simulink library "VISMODAL_MASTER"  (Simulink 8.6)
settings: Solver=VariableStepAuto  StartTime=0.0  StopTime=10.0  RelTol=1e-3
libraries: VIS_LIB x140, cdsFilt x34, cdsMuxMatrix x6, VISMODAL_MASTER x1
(part 4 of 5)

== system VISMODAL_MASTER/ITMY/SUM_GAS ==
  note: #DAQ Channels
      |
      | M1_OUT 256
      | M2_OUT 256
      | M3_OUT 256
      | M4_OUT 256
      | M5_OUT 256
  M1_IN : Inport
  M2_IN : Inport  Port=2
  M3_IN : Inport  Port=3
  M4_IN : Inport  Port=4
  M5_IN : Inport  Port=5
  M1 : cdsFilt/Subsystem  Tag=cdsFilt  Description=|
      | Purpose:                                                                                                                                                                                                                                  
      | Standard CDS IIR filter module.                                                                                                                                                                                                           
      |                                                                                                                                                                                                                                           
      | Operation:                                                                                                                                                                                                                                
      | Consists of 10 second order section IIR filters, plus a ramped gain stage. In FE code, also provides pre-defined test points and excitation channel inputs. The filter coefficients are defined in the LIGO system using the 'foton' tool.
      |                                                                                                                                                                                                                                           
      | Usage:                                                                                                                                                                                                                                    
      | Name the part with the desired filter module name.
      settings: AttributesFormatString=%<Tag>
  M2 : cdsFilt/Subsystem  Tag=cdsFilt  Description=|
      | Purpose:                                                                                                                                                                                                                                  
      | Standard CDS IIR filter module.                                                                                                                                                                                                           
      |                                                                                                                                                                                                                                           
      | Operation:                                                                                                                                                                                                                                
      | Consists of 10 second order section IIR filters, plus a ramped gain stage. In FE code, also provides pre-defined test points and excitation channel inputs. The filter coefficients are defined in the LIGO system using the 'foton' tool.
      |                                                                                                                                                                                                                                           
      | Usage:                                                                                                                                                                                                                                    
      | Name the part with the desired filter module name.
      settings: AttributesFormatString=%<Tag>
  M3 : cdsFilt/Subsystem  Tag=cdsFilt  Description=|
      | Purpose:                                                                                                                                                                                                                                  
      | Standard CDS IIR filter module.                                                                                                                                                                                                           
      |                                                                                                                                                                                                                                           
      | Operation:                                                                                                                                                                                                                                
      | Consists of 10 second order section IIR filters, plus a ramped gain stage. In FE code, also provides pre-defined test points and excitation channel inputs. The filter coefficients are defined in the LIGO system using the 'foton' tool.
      |                                                                                                                                                                                                                                           
      | Usage:                                                                                                                                                                                                                                    
      | Name the part with the desired filter module name.
      settings: AttributesFormatString=%<Tag>
  M4 : cdsFilt/Subsystem  Tag=cdsFilt  Description=|
      | Purpose:                                                                                                                                                                                                                                  
      | Standard CDS IIR filter module.                                                                                                                                                                                                           
      |                                                                                                                                                                                                                                           
      | Operation:                                                                                                                                                                                                                                
      | Consists of 10 second order section IIR filters, plus a ramped gain stage. In FE code, also provides pre-defined test points and excitation channel inputs. The filter coefficients are defined in the LIGO system using the 'foton' tool.
      |                                                                                                                                                                                                                                           
      | Usage:                                                                                                                                                                                                                                    
      | Name the part with the desired filter module name.
      settings: AttributesFormatString=%<Tag>
  M5 : cdsFilt/Subsystem  Tag=cdsFilt  Description=|
      | Purpose:                                                                                                                                                                                                                                  
      | Standard CDS IIR filter module.                                                                                                                                                                                                           
      |                                                                                                                                                                                                                                           
      | Operation:                                                                                                                                                                                                                                
      | Consists of 10 second order section IIR filters, plus a ramped gain stage. In FE code, also provides pre-defined test points and excitation channel inputs. The filter coefficients are defined in the LIGO system using the 'foton' tool.
      |                                                                                                                                                                                                                                           
      | Usage:                                                                                                                                                                                                                                    
      | Name the part with the desired filter module name.
      settings: AttributesFormatString=%<Tag>
  M1_OUT : Outport
  M2_OUT : Outport  Port=2
  M3_OUT : Outport  Port=3
  M4_OUT : Outport  Port=4
  M5_OUT : Outport  Port=5
  wires:
  M3/1 -> M3_OUT/1
  M2/1 -> M2_OUT/1
  M4/1 -> M4_OUT/1
  M5/1 -> M5_OUT/1
  M1/1 -> M1_OUT/1
  M1_IN/1 -> M1/1
  M2_IN/1 -> M2/1
  M3_IN/1 -> M3/1
  M4_IN/1 -> M4/1
  M5_IN/1 -> M5/1

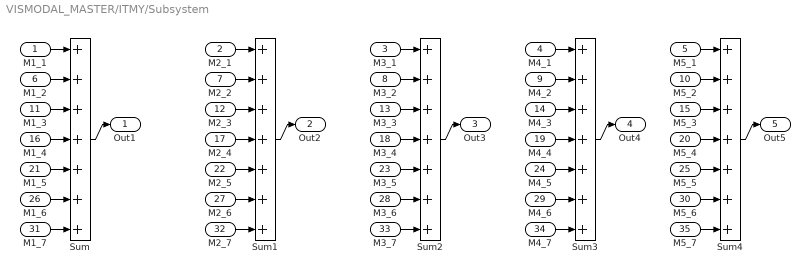
== system VISMODAL_MASTER/ITMY/Subsystem ==
  M1_1 : Inport
  M2_1 : Inport  Port=2
  M3_1 : Inport  Port=3
  M4_1 : Inport  Port=4
  M5_1 : Inport  Port=5
  M1_2 : Inport  Port=6
  M2_2 : Inport  Port=7
  M3_2 : Inport  Port=8
  M4_2 : Inport  Port=9
  M5_2 : Inport  Port=10
  M1_3 : Inport  Port=11
  M2_3 : Inport  Port=12
  M3_3 : Inport  Port=13
  M4_3 : Inport  Port=14
  M5_3 : Inport  Port=15
  M1_4 : Inport  Port=16
  M2_4 : Inport  Port=17
  M3_4 : Inport  Port=18
  M4_4 : Inport  Port=19
  M5_4 : Inport  Port=20
  M1_5 : Inport  Port=21
  M2_5 : Inport  Port=22
  M3_5 : Inport  Port=23
  M4_5 : Inport  Port=24
  M5_5 : Inport  Port=25
  M1_6 : Inport  Port=26
  M2_6 : Inport  Port=27
  M3_6 : Inport  Port=28
  M4_6 : Inport  Port=29
  M5_6 : Inport  Port=30
  M1_7 : Inport  Port=31
  M2_7 : Inport  Port=32
  M3_7 : Inport  Port=33
  M4_7 : Inport  Port=34
  M5_7 : Inport  Port=35
  Sum{,1..4} (5 alike) : Sum  Inputs=+++++++
  Out1 : Outport
  Out2 : Outport  Port=2
  Out3 : Outport  Port=3
  Out4 : Outport  Port=4
  Out5 : Outport  Port=5
  wires:
  M1_1/1 -> Sum/1
  Sum/1 -> Out1/1
  M2_1/1 -> Sum1/1
  Sum1/1 -> Out2/1
  M3_1/1 -> Sum2/1
  Sum2/1 -> Out3/1
  M4_1/1 -> Sum3/1
  Sum3/1 -> Out4/1
  M5_1/1 -> Sum4/1
  Sum4/1 -> Out5/1
  M1_2/1 -> Sum/2
  M2_2/1 -> Sum1/2
  M3_2/1 -> Sum2/2
  M4_2/1 -> Sum3/2
  M5_2/1 -> Sum4/2
  M1_3/1 -> Sum/3
  M2_3/1 -> Sum1/3
  M3_3/1 -> Sum2/3
  M4_3/1 -> Sum3/3
  M5_3/1 -> Sum4/3
  M1_4/1 -> Sum/4
  M2_4/1 -> Sum1/4
  M3_4/1 -> Sum2/4
  M4_4/1 -> Sum3/4
  M5_4/1 -> Sum4/4
  M1_5/1 -> Sum/5
  M2_5/1 -> Sum1/5
  M3_5/1 -> Sum2/5
  M4_5/1 -> Sum3/5
  M5_5/1 -> Sum4/5
  M1_6/1 -> Sum/6
  M2_6/1 -> Sum1/6
  M3_6/1 -> Sum2/6
  M4_6/1 -> Sum3/6
  M5_6/1 -> Sum4/6
  M5_7/1 -> Sum4/7
  M4_7/1 -> Sum3/7
  M3_7/1 -> Sum2/7
  M2_7/1 -> Sum1/7
  M1_7/1 -> Sum/7

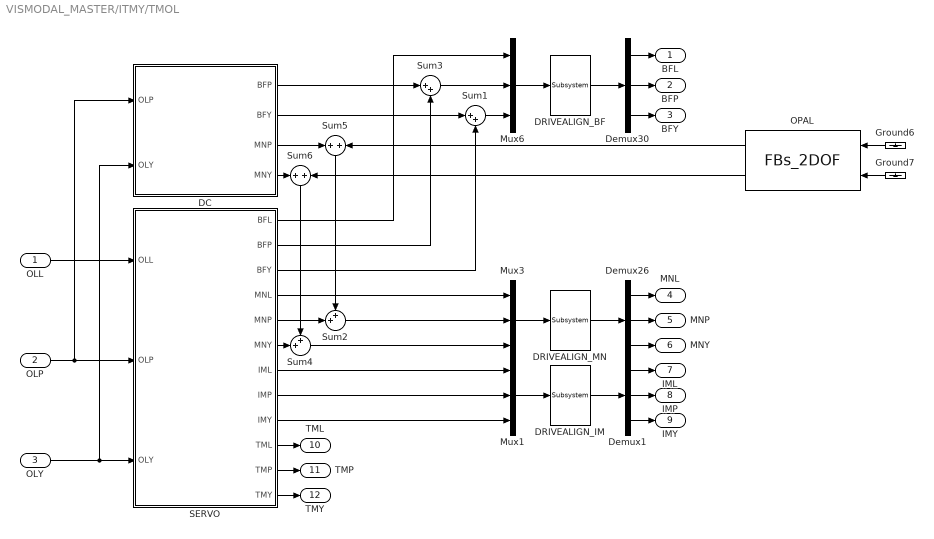
== system VISMODAL_MASTER/ITMY/TMOL ==
  OLL : Inport
  OLP : Inport  Port=2
  OLY : Inport  Port=3
  DC : Subsystem
  DRIVEALIGN_BF : cdsMuxMatrix/Subsystem  Tag=cdsMuxMatrix  Description=Any size matrix. Inputs and outputs must be connected using Mux and Demux parts.
      settings: AttributesFormatString=%<Tag>
  DRIVEALIGN_IM : cdsMuxMatrix/Subsystem  Tag=cdsMuxMatrix  Description=Any size matrix. Inputs and outputs must be connected using Mux and Demux parts.
      settings: AttributesFormatString=%<Tag>
  DRIVEALIGN_MN : cdsMuxMatrix/Subsystem  Tag=cdsMuxMatrix  Description=Any size matrix. Inputs and outputs must be connected using Mux and Demux parts.
      settings: AttributesFormatString=%<Tag>
  Demux1 : Demux  Outputs=3
  Demux26 : Demux  Outputs=3
  Demux30 : Demux  Outputs=3
  Ground6 : Ground
  Ground7 : Ground
  Mux1 : Mux  Inputs=3
  Mux3 : Mux  Inputs=3
  Mux6 : Mux  Inputs=3
  OPAL : VIS_LIB/UTILs/FBs_2DOF
  SERVO : Subsystem
  Sum1 : Sum  Inputs=|++
  Sum2 : Sum  Inputs=++|
  Sum3 : Sum  Inputs=|++
  Sum4 : Sum  Inputs=++|
  Sum5 : Sum
  Sum6 : Sum
  BFL : Outport
  BFP : Outport  Port=2
  BFY : Outport  Port=3
  MNL : Outport  Port=4
  MNP : Outport  Port=5
  MNY : Outport  Port=6
  IML : Outport  Port=7
  IMP : Outport  Port=8
  IMY : Outport  Port=9
  TML : Outport  Port=10
  TMP : Outport  Port=11
  TMY : Outport  Port=12
  wires:
  Mux3/1 -> DRIVEALIGN_MN/1
  DRIVEALIGN_MN/1 -> Demux26/1
  Mux6/1 -> DRIVEALIGN_BF/1
  DRIVEALIGN_BF/1 -> Demux30/1
  Demux30/1 -> BFL/1
  Demux30/2 -> BFP/1
  Demux26/1 -> MNL/1
  Demux26/2 -> MNP/1
  SERVO/1(BFL) -> Mux6/1
  Sum3/1 -> Mux6/2
  SERVO/2(BFP) -> Sum3/2
  DC/1(BFP) -> Sum3/1
  Sum1/1 -> Mux6/3
  DC/2(BFY) -> Sum1/1
  SERVO/3(BFY) -> Sum1/2
  SERVO/4(MNL) -> Mux3/1
  Sum2/1 -> Mux3/2
  SERVO/5(MNP) -> Sum2/2
  SERVO/6(MNY) -> Sum4/2
  Sum4/1 -> Mux3/3
  Demux30/3 -> BFY/1
  Demux26/3 -> MNY/1
  Mux1/1 -> DRIVEALIGN_IM/1
  DRIVEALIGN_IM/1 -> Demux1/1
  Demux1/1 -> IML/1
  Demux1/2 -> IMP/1
  SERVO/7(IML) -> Mux1/1
  SERVO/8(IMP) -> Mux1/2
  SERVO/9(IMY) -> Mux1/3
  Demux1/3 -> IMY/1
  SERVO/10(TML) -> TML/1
  SERVO/11(TMP) -> TMP/1
  SERVO/12(TMY) -> TMY/1
  DC/3(MNP) -> Sum5/1
  Sum5/1 -> Sum2/1
  DC/4(MNY) -> Sum6/1
  Sum6/1 -> Sum4/1
  OLL/1 -> SERVO/1(OLL)
  OLP/1 -> DC/1(OLP), SERVO/2(OLP)
  OLY/1 -> DC/2(OLY), SERVO/3(OLY)
  Ground6/1 -> OPAL/1
  Ground7/1 -> OPAL/2
  OPAL/2 -> Sum6/2
  OPAL/1 -> Sum5/2

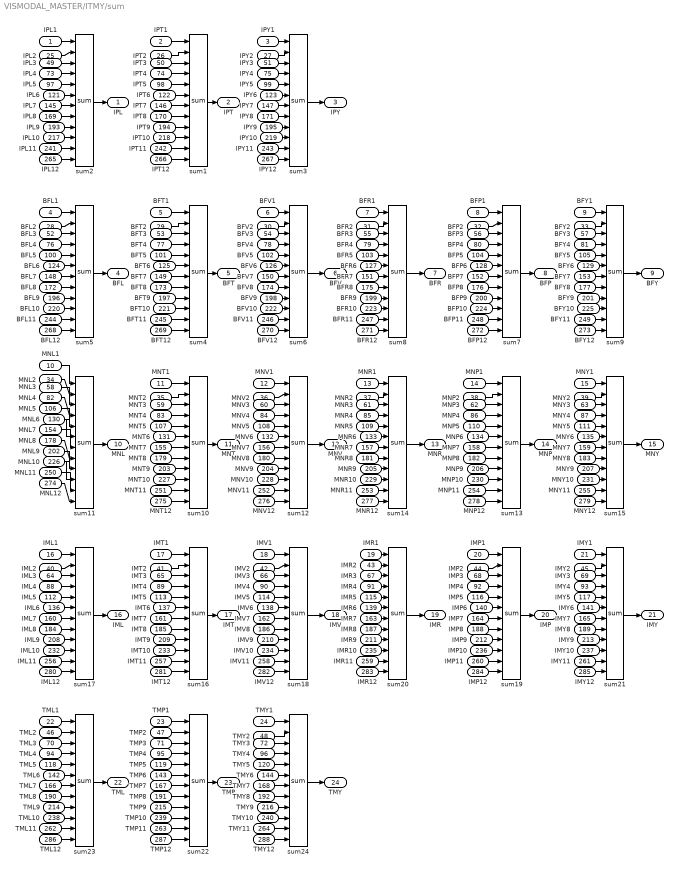
== system VISMODAL_MASTER/ITMY/sum ==
  IPL1 : Inport
  IPT1 : Inport  Port=2
  IPY1 : Inport  Port=3
  BFL1 : Inport  Port=4
  BFT1 : Inport  Port=5
  BFV1 : Inport  Port=6
  BFR1 : Inport  Port=7
  BFP1 : Inport  Port=8
  BFY1 : Inport  Port=9
  MNL1 : Inport  Port=10
  MNT1 : Inport  Port=11
  MNV1 : Inport  Port=12
  MNR1 : Inport  Port=13
  MNP1 : Inport  Port=14
  MNY1 : Inport  Port=15
  IML1 : Inport  Port=16
  IMT1 : Inport  Port=17
  IMV1 : Inport  Port=18
  IMR1 : Inport  Port=19
  IMP1 : Inport  Port=20
  IMY1 : Inport  Port=21
  TML1 : Inport  Port=22
  TMP1 : Inport  Port=23
  TMY1 : Inport  Port=24
  IPL2 : Inport  Port=25
  IPT2 : Inport  Port=26
  IPY2 : Inport  Port=27
  BFL2 : Inport  Port=28
  BFT2 : Inport  Port=29
  BFV2 : Inport  Port=30
  BFR2 : Inport  Port=31
  BFP2 : Inport  Port=32
  BFY2 : Inport  Port=33
  MNL2 : Inport  Port=34
  MNT2 : Inport  Port=35
  MNV2 : Inport  Port=36
  MNR2 : Inport  Port=37
  MNP2 : Inport  Port=38
  MNY2 : Inport  Port=39
  IML2 : Inport  Port=40
  IMT2 : Inport  Port=41
  IMV2 : Inport  Port=42
  IMR2 : Inport  Port=43
  IMP2 : Inport  Port=44
  IMY2 : Inport  Port=45
  TML2 : Inport  Port=46
  TMP2 : Inport  Port=47
  TMY2 : Inport  Port=48
  IPL3 : Inport  Port=49
  IPT3 : Inport  Port=50
  IPY3 : Inport  Port=51
  BFL3 : Inport  Port=52
  BFT3 : Inport  Port=53
  BFV3 : Inport  Port=54
  BFR3 : Inport  Port=55
  BFP3 : Inport  Port=56
  BFY3 : Inport  Port=57
  MNL3 : Inport  Port=58
  MNT3 : Inport  Port=59
  MNV3 : Inport  Port=60
  MNR3 : Inport  Port=61
  MNP3 : Inport  Port=62
  MNY3 : Inport  Port=63
  IML3 : Inport  Port=64
  IMT3 : Inport  Port=65
  IMV3 : Inport  Port=66
  IMR3 : Inport  Port=67
  IMP3 : Inport  Port=68
  IMY3 : Inport  Port=69
  TML3 : Inport  Port=70
  TMP3 : Inport  Port=71
  TMY3 : Inport  Port=72
  IPL4 : Inport  Port=73
  IPT4 : Inport  Port=74
  IPY4 : Inport  Port=75
  BFL4 : Inport  Port=76
  BFT4 : Inport  Port=77
  BFV4 : Inport  Port=78
  BFR4 : Inport  Port=79
  BFP4 : Inport  Port=80
  BFY4 : Inport  Port=81
  MNL4 : Inport  Port=82
  MNT4 : Inport  Port=83
  MNV4 : Inport  Port=84
  MNR4 : Inport  Port=85
  MNP4 : Inport  Port=86
  MNY4 : Inport  Port=87
  IML4 : Inport  Port=88
  IMT4 : Inport  Port=89
  IMV4 : Inport  Port=90
  IMR4 : Inport  Port=91
  IMP4 : Inport  Port=92
  IMY4 : Inport  Port=93
  TML4 : Inport  Port=94
  TMP4 : Inport  Port=95
  TMY4 : Inport  Port=96
  IPL5 : Inport  Port=97
  IPT5 : Inport  Port=98
  IPY5 : Inport  Port=99
  BFL5 : Inport  Port=100
  BFT5 : Inport  Port=101
  BFV5 : Inport  Port=102
  BFR5 : Inport  Port=103
  BFP5 : Inport  Port=104
  BFY5 : Inport  Port=105
  MNL5 : Inport  Port=106
  MNT5 : Inport  Port=107
  MNV5 : Inport  Port=108
  MNR5 : Inport  Port=109
  MNP5 : Inport  Port=110
  MNY5 : Inport  Port=111
  IML5 : Inport  Port=112
  IMT5 : Inport  Port=113
  IMV5 : Inport  Port=114
  IMR5 : Inport  Port=115
  IMP5 : Inport  Port=116
  IMY5 : Inport  Port=117
  TML5 : Inport  Port=118
  TMP5 : Inport  Port=119
  TMY5 : Inport  Port=120
  IPL6 : Inport  Port=121
  IPT6 : Inport  Port=122
  IPY6 : Inport  Port=123
  BFL6 : Inport  Port=124
  BFT6 : Inport  Port=125
  BFV6 : Inport  Port=126
  BFR6 : Inport  Port=127
  BFP6 : Inport  Port=128
  BFY6 : Inport  Port=129
  MNL6 : Inport  Port=130
  MNT6 : Inport  Port=131
  MNV6 : Inport  Port=132
  MNR6 : Inport  Port=133
  MNP6 : Inport  Port=134
  MNY6 : Inport  Port=135
  IML6 : Inport  Port=136
  IMT6 : Inport  Port=137
  IMV6 : Inport  Port=138
  IMR6 : Inport  Port=139
  IMP6 : Inport  Port=140
  IMY6 : Inport  Port=141
  TML6 : Inport  Port=142
  TMP6 : Inport  Port=143
  TMY6 : Inport  Port=144
  IPL7 : Inport  Port=145
  IPT7 : Inport  Port=146
  IPY7 : Inport  Port=147
  BFL7 : Inport  Port=148
  BFT7 : Inport  Port=149
  BFV7 : Inport  Port=150
  BFR7 : Inport  Port=151
  BFP7 : Inport  Port=152
  BFY7 : Inport  Port=153
  MNL7 : Inport  Port=154
  MNT7 : Inport  Port=155
  MNV7 : Inport  Port=156
  MNR7 : Inport  Port=157
  MNP7 : Inport  Port=158
  MNY7 : Inport  Port=159
  IML7 : Inport  Port=160
  IMT7 : Inport  Port=161
  IMV7 : Inport  Port=162
  IMR7 : Inport  Port=163
  IMP7 : Inport  Port=164
  IMY7 : Inport  Port=165
  TML7 : Inport  Port=166
  TMP7 : Inport  Port=167
  TMY7 : Inport  Port=168
  IPL8 : Inport  Port=169
  IPT8 : Inport  Port=170
  IPY8 : Inport  Port=171
  BFL8 : Inport  Port=172
  BFT8 : Inport  Port=173
  BFV8 : Inport  Port=174
  BFR8 : Inport  Port=175
  BFP8 : Inport  Port=176
  BFY8 : Inport  Port=177
  MNL8 : Inport  Port=178
  MNT8 : Inport  Port=179
  MNV8 : Inport  Port=180
  MNR8 : Inport  Port=181
  MNP8 : Inport  Port=182
  MNY8 : Inport  Port=183
  IML8 : Inport  Port=184
  IMT8 : Inport  Port=185
  IMV8 : Inport  Port=186
  IMR8 : Inport  Port=187
  IMP8 : Inport  Port=188
  IMY8 : Inport  Port=189
  TML8 : Inport  Port=190
  TMP8 : Inport  Port=191
  TMY8 : Inport  Port=192
  IPL9 : Inport  Port=193
  IPT9 : Inport  Port=194
  IPY9 : Inport  Port=195
  BFL9 : Inport  Port=196
  BFT9 : Inport  Port=197
  BFV9 : Inport  Port=198
  BFR9 : Inport  Port=199
  BFP9 : Inport  Port=200
  BFY9 : Inport  Port=201
  MNL9 : Inport  Port=202
  MNT9 : Inport  Port=203
  MNV9 : Inport  Port=204
  MNR9 : Inport  Port=205
  MNP9 : Inport  Port=206
  MNY9 : Inport  Port=207
  IML9 : Inport  Port=208
  IMT9 : Inport  Port=209
  IMV9 : Inport  Port=210
  IMR9 : Inport  Port=211
  IMP9 : Inport  Port=212
  IMY9 : Inport  Port=213
  TML9 : Inport  Port=214
  TMP9 : Inport  Port=215
  TMY9 : Inport  Port=216
  IPL10 : Inport  Port=217
  IPT10 : Inport  Port=218
  IPY10 : Inport  Port=219
  BFL10 : Inport  Port=220
  BFT10 : Inport  Port=221
  BFV10 : Inport  Port=222
  BFR10 : Inport  Port=223
  BFP10 : Inport  Port=224
  BFY10 : Inport  Port=225
  MNL10 : Inport  Port=226
  MNT10 : Inport  Port=227
  MNV10 : Inport  Port=228
  MNR10 : Inport  Port=229
  MNP10 : Inport  Port=230
  MNY10 : Inport  Port=231
  IML10 : Inport  Port=232
  IMT10 : Inport  Port=233
  IMV10 : Inport  Port=234
  IMR10 : Inport  Port=235
  IMP10 : Inport  Port=236
  IMY10 : Inport  Port=237
  TML10 : Inport  Port=238
  TMP10 : Inport  Port=239
  TMY10 : Inport  Port=240
  IPL11 : Inport  Port=241
  IPT11 : Inport  Port=242
  IPY11 : Inport  Port=243
  BFL11 : Inport  Port=244
  BFT11 : Inport  Port=245
  BFV11 : Inport  Port=246
  BFR11 : Inport  Port=247
  BFP11 : Inport  Port=248
  BFY11 : Inport  Port=249
  MNL11 : Inport  Port=250
  MNT11 : Inport  Port=251
  MNV11 : Inport  Port=252
  MNR11 : Inport  Port=253
  MNP11 : Inport  Port=254
  MNY11 : Inport  Port=255
  IML11 : Inport  Port=256
  IMT11 : Inport  Port=257
  IMV11 : Inport  Port=258
  IMR11 : Inport  Port=259
  IMP11 : Inport  Port=260
  IMY11 : Inport  Port=261
  TML11 : Inport  Port=262
  TMP11 : Inport  Port=263
  TMY11 : Inport  Port=264
  IPL12 : Inport  Port=265
  IPT12 : Inport  Port=266
  IPY12 : Inport  Port=267
  BFL12 : Inport  Port=268
  BFT12 : Inport  Port=269
  BFV12 : Inport  Port=270
  BFR12 : Inport  Port=271
  BFP12 : Inport  Port=272
  BFY12 : Inport  Port=273
  MNL12 : Inport  Port=274
  MNT12 : Inport  Port=275
  MNV12 : Inport  Port=276
  MNR12 : Inport  Port=277
  MNP12 : Inport  Port=278
  MNY12 : Inport  Port=279
  IML12 : Inport  Port=280
  IMT12 : Inport  Port=281
  IMV12 : Inport  Port=282
  IMR12 : Inport  Port=283
  IMP12 : Inport  Port=284
  IMY12 : Inport  Port=285
  TML12 : Inport  Port=286
  TMP12 : Inport  Port=287
  TMY12 : Inport  Port=288
  sum{1..24} (24 alike) : VIS_LIB/MODAL/sum
  IPL : Outport
  IPT : Outport  Port=2
  IPY : Outport  Port=3
  BFL : Outport  Port=4
  BFT : Outport  Port=5
  BFV : Outport  Port=6
  BFR : Outport  Port=7
  BFP : Outport  Port=8
  BFY : Outport  Port=9
  MNL : Outport  Port=10
  MNT : Outport  Port=11
  MNV : Outport  Port=12
  MNR : Outport  Port=13
  MNP : Outport  Port=14
  MNY : Outport  Port=15
  IML : Outport  Port=16
  IMT : Outport  Port=17
  IMV : Outport  Port=18
  IMR : Outport  Port=19
  IMP : Outport  Port=20
  IMY : Outport  Port=21
  TML : Outport  Port=22
  TMP : Outport  Port=23
  TMY : Outport  Port=24
  wires:
  IPT2/1 -> sum1/2
  IPT1/1 -> sum1/1
  IPL1/1 -> sum2/1
  IPL2/1 -> sum2/2
  IPY1/1 -> sum3/1
  IPY2/1 -> sum3/2
  BFT1/1 -> sum4/1
  BFT2/1 -> sum4/2
  BFL1/1 -> sum5/1
  BFL2/1 -> sum5/2
  BFV1/1 -> sum6/1
  BFV2/1 -> sum6/2
  BFR1/1 -> sum8/1
  BFR2/1 -> sum8/2
  BFP1/1 -> sum7/1
  BFP2/1 -> sum7/2
  BFY1/1 -> sum9/1
  BFY2/1 -> sum9/2
  MNT1/1 -> sum10/1
  MNT2/1 -> sum10/2
  MNL1/1 -> sum11/1
  MNL2/1 -> sum11/2
  MNV1/1 -> sum12/1
  MNV2/1 -> sum12/2
  MNR1/1 -> sum14/1
  MNR2/1 -> sum14/2
  MNP1/1 -> sum13/1
  MNP2/1 -> sum13/2
  MNY1/1 -> sum15/1
  MNY2/1 -> sum15/2
  IMT1/1 -> sum16/1
  IMT2/1 -> sum16/2
  IML1/1 -> sum17/1
  IML2/1 -> sum17/2
  IMV1/1 -> sum18/1
  IMV2/1 -> sum18/2
  IMP1/1 -> sum19/1
  IMP2/1 -> sum19/2
  IMY1/1 -> sum21/1
  IMY2/1 -> sum21/2
  TML2/1 -> sum23/2
  TML1/1 -> sum23/1
  TMP1/1 -> sum22/1
  TMP2/1 -> sum22/2
  TMY1/1 -> sum24/1
  TMY2/1 -> sum24/2
  sum24/1 -> TMY/1
  sum22/1 -> TMP/1
  sum23/1 -> TML/1
  sum17/1 -> IML/1
  sum16/1 -> IMT/1
  sum18/1 -> IMV/1
  sum20/1 -> IMR/1
  sum19/1 -> IMP/1
  sum21/1 -> IMY/1
  sum3/1 -> IPY/1
  sum1/1 -> IPT/1
  sum4/1 -> BFT/1
  sum6/1 -> BFV/1
  sum12/1 -> MNV/1
  sum14/1 -> MNR/1
  sum8/1 -> BFR/1
  sum7/1 -> BFP/1
  sum9/1 -> BFY/1
  sum15/1 -> MNY/1
  sum13/1 -> MNP/1
  sum10/1 -> MNT/1
  sum11/1 -> MNL/1
  sum5/1 -> BFL/1
  sum2/1 -> IPL/1
  IPT3/1 -> sum1/3
  IPL3/1 -> sum2/3
  IPY3/1 -> sum3/3
  BFT3/1 -> sum4/3
  BFL3/1 -> sum5/3
  BFV3/1 -> sum6/3
  BFR3/1 -> sum8/3
  BFP3/1 -> sum7/3
  BFY3/1 -> sum9/3
  MNT3/1 -> sum10/3
  MNL3/1 -> sum11/3
  MNV3/1 -> sum12/3
  MNR3/1 -> sum14/3
  MNP3/1 -> sum13/3
  MNY3/1 -> sum15/3
  IMT3/1 -> sum16/3
  IML3/1 -> sum17/3
  IMV3/1 -> sum18/3
  IMP3/1 -> sum19/3
  IMY3/1 -> sum21/3
  TML3/1 -> sum23/3
  TMP3/1 -> sum22/3
  TMY3/1 -> sum24/3
  IPT4/1 -> sum1/4
  IPL4/1 -> sum2/4
  IPY4/1 -> sum3/4
  BFT4/1 -> sum4/4
  BFL4/1 -> sum5/4
  BFV4/1 -> sum6/4
  BFR4/1 -> sum8/4
  BFP4/1 -> sum7/4
  BFY4/1 -> sum9/4
  MNT4/1 -> sum10/4
  MNL4/1 -> sum11/4
  MNV4/1 -> sum12/4
  MNR4/1 -> sum14/4
  MNP4/1 -> sum13/4
  MNY4/1 -> sum15/4
  IMT4/1 -> sum16/4
  IML4/1 -> sum17/4
  IMV4/1 -> sum18/4
  IMP4/1 -> sum19/4
  IMY4/1 -> sum21/4
  TML4/1 -> sum23/4
  TMP4/1 -> sum22/4
  TMY4/1 -> sum24/4
  IPT5/1 -> sum1/5
  IPL5/1 -> sum2/5
  IPY5/1 -> sum3/5
  BFT5/1 -> sum4/5
  BFL5/1 -> sum5/5
  BFV5/1 -> sum6/5
  BFR5/1 -> sum8/5
  BFP5/1 -> sum7/5
  BFY5/1 -> sum9/5
  MNT5/1 -> sum10/5
  MNL5/1 -> sum11/5
  MNV5/1 -> sum12/5
  MNR5/1 -> sum14/5
  MNP5/1 -> sum13/5
  MNY5/1 -> sum15/5
  IMT5/1 -> sum16/5
  IML5/1 -> sum17/5
  IMV5/1 -> sum18/5
  IMP5/1 -> sum19/5
  IMY5/1 -> sum21/5
  TML5/1 -> sum23/5
  TMP5/1 -> sum22/5
  TMY5/1 -> sum24/5
  IPT6/1 -> sum1/6
  IPL6/1 -> sum2/6
  IPY6/1 -> sum3/6
  BFT6/1 -> sum4/6
  BFL6/1 -> sum5/6
  BFV6/1 -> sum6/6
  BFR6/1 -> sum8/6
  BFP6/1 -> sum7/6
  BFY6/1 -> sum9/6
  MNT6/1 -> sum10/6
  MNL6/1 -> sum11/6
  MNV6/1 -> sum12/6
  MNR6/1 -> sum14/6
  MNP6/1 -> sum13/6
  MNY6/1 -> sum15/6
  IMT6/1 -> sum16/6
  IML6/1 -> sum17/6
  IMV6/1 -> sum18/6
  IMP6/1 -> sum19/6
  IMY6/1 -> sum21/6
  TML6/1 -> sum23/6
  TMP6/1 -> sum22/6
  TMY6/1 -> sum24/6
  IPT7/1 -> sum1/7
  IPL7/1 -> sum2/7
  IPY7/1 -> sum3/7
  BFT7/1 -> sum4/7
  BFL7/1 -> sum5/7
  BFV7/1 -> sum6/7
  BFR7/1 -> sum8/7
  BFP7/1 -> sum7/7
  BFY7/1 -> sum9/7
  MNT7/1 -> sum10/7
  MNL7/1 -> sum11/7
  MNV7/1 -> sum12/7
  MNR7/1 -> sum14/7
  MNP7/1 -> sum13/7
  MNY7/1 -> sum15/7
  IMT7/1 -> sum16/7
  IML7/1 -> sum17/7
  IMV7/1 -> sum18/7
  IMP7/1 -> sum19/7
  IMY7/1 -> sum21/7
  TML7/1 -> sum23/7
  TMP7/1 -> sum22/7
  TMY7/1 -> sum24/7
  IPT8/1 -> sum1/8
  IPL8/1 -> sum2/8
  IPY8/1 -> sum3/8
  BFT8/1 -> sum4/8
  BFL8/1 -> sum5/8
  BFV8/1 -> sum6/8
  BFR8/1 -> sum8/8
  BFP8/1 -> sum7/8
  BFY8/1 -> sum9/8
  MNT8/1 -> sum10/8
  MNL8/1 -> sum11/8
  MNV8/1 -> sum12/8
  MNR8/1 -> sum14/8
  MNP8/1 -> sum13/8
  MNY8/1 -> sum15/8
  IMT8/1 -> sum16/8
  IML8/1 -> sum17/8
  IMV8/1 -> sum18/8
  IMP8/1 -> sum19/8
  IMY8/1 -> sum21/8
  TML8/1 -> sum23/8
  TMP8/1 -> sum22/8
  TMY8/1 -> sum24/8
  IPT9/1 -> sum1/9
  IPL9/1 -> sum2/9
  IPY9/1 -> sum3/9
  BFT9/1 -> sum4/9
  BFL9/1 -> sum5/9
  BFV9/1 -> sum6/9
  BFR9/1 -> sum8/9
  BFP9/1 -> sum7/9
  BFY9/1 -> sum9/9
  MNT9/1 -> sum10/9
  MNL9/1 -> sum11/9
  MNV9/1 -> sum12/9
  MNR9/1 -> sum14/9
  MNP9/1 -> sum13/9
  MNY9/1 -> sum15/9
  IMT9/1 -> sum16/9
  IML9/1 -> sum17/9
  IMV9/1 -> sum18/9
  IMP9/1 -> sum19/9
  IMY9/1 -> sum21/9
  TML9/1 -> sum23/9
  TMP9/1 -> sum22/9
  TMY9/1 -> sum24/9
  IPT10/1 -> sum1/10
  IPL10/1 -> sum2/10
  IPY10/1 -> sum3/10
  BFT10/1 -> sum4/10
  BFL10/1 -> sum5/10
  BFV10/1 -> sum6/10
  BFR10/1 -> sum8/10
  BFP10/1 -> sum7/10
  BFY10/1 -> sum9/10
  MNT10/1 -> sum10/10
  MNL10/1 -> sum11/10
  MNV10/1 -> sum12/10
  MNR10/1 -> sum14/10
  MNP10/1 -> sum13/10
  MNY10/1 -> sum15/10
  IMT10/1 -> sum16/10
  IML10/1 -> sum17/10
  IMV10/1 -> sum18/10
  IMP10/1 -> sum19/10
  IMY10/1 -> sum21/10
  TML10/1 -> sum23/10
  TMP10/1 -> sum22/10
  TMY10/1 -> sum24/10
  IPT11/1 -> sum1/11
  IPL11/1 -> sum2/11
  IPY11/1 -> sum3/11
  BFT11/1 -> sum4/11
  BFL11/1 -> sum5/11
  BFV11/1 -> sum6/11
  BFR11/1 -> sum8/11
  BFP11/1 -> sum7/11
  BFY11/1 -> sum9/11
  MNT11/1 -> sum10/11
  MNL11/1 -> sum11/11
  MNV11/1 -> sum12/11
  MNR11/1 -> sum14/11
  MNP11/1 -> sum13/11
  MNY11/1 -> sum15/11
  IMT11/1 -> sum16/11
  IML11/1 -> sum17/11
  IMV11/1 -> sum18/11
  IMP11/1 -> sum19/11
  IMY11/1 -> sum21/11
  TML11/1 -> sum23/11
  TMP11/1 -> sum22/11
  TMY11/1 -> sum24/11
  IPT12/1 -> sum1/12
  IPL12/1 -> sum2/12
  IPY12/1 -> sum3/12
  BFT12/1 -> sum4/12
  BFL12/1 -> sum5/12
  BFV12/1 -> sum6/12
  BFR12/1 -> sum8/12
  BFP12/1 -> sum7/12
  BFY12/1 -> sum9/12
  MNT12/1 -> sum10/12
  MNL12/1 -> sum11/12
  MNV12/1 -> sum12/12
  MNR12/1 -> sum14/12
  MNP12/1 -> sum13/12
  MNY12/1 -> sum15/12
  IMT12/1 -> sum16/12
  IML12/1 -> sum17/12
  IMV12/1 -> sum18/12
  IMP12/1 -> sum19/12
  IMY12/1 -> sum21/12
  TML12/1 -> sum23/12
  TMP12/1 -> sum22/12
  TMY12/1 -> sum24/12
  IMR12/1 -> sum20/12
  IMR11/1 -> sum20/11
  IMR10/1 -> sum20/10
  IMR9/1 -> sum20/9
  IMR8/1 -> sum20/8
  IMR7/1 -> sum20/7
  IMR6/1 -> sum20/6
  IMR5/1 -> sum20/5
  IMR4/1 -> sum20/4
  IMR3/1 -> sum20/3
  IMR2/1 -> sum20/2
  IMR1/1 -> sum20/1

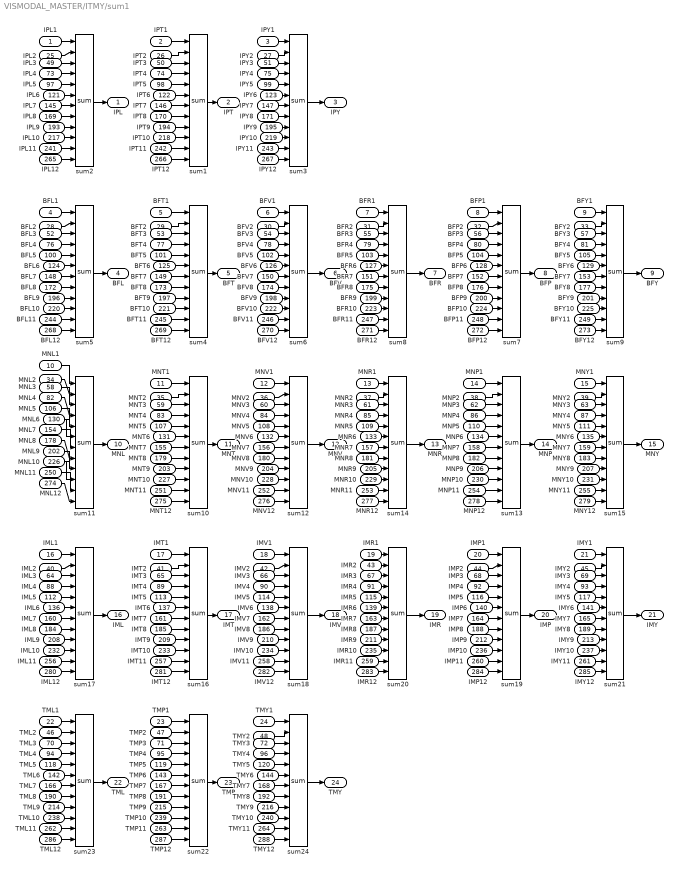
== system VISMODAL_MASTER/ITMY/sum1 ==
  IPL1 : Inport
  IPT1 : Inport  Port=2
  IPY1 : Inport  Port=3
  BFL1 : Inport  Port=4
  BFT1 : Inport  Port=5
  BFV1 : Inport  Port=6
  BFR1 : Inport  Port=7
  BFP1 : Inport  Port=8
  BFY1 : Inport  Port=9
  MNL1 : Inport  Port=10
  MNT1 : Inport  Port=11
  MNV1 : Inport  Port=12
  MNR1 : Inport  Port=13
  MNP1 : Inport  Port=14
  MNY1 : Inport  Port=15
  IML1 : Inport  Port=16
  IMT1 : Inport  Port=17
  IMV1 : Inport  Port=18
  IMR1 : Inport  Port=19
  IMP1 : Inport  Port=20
  IMY1 : Inport  Port=21
  TML1 : Inport  Port=22
  TMP1 : Inport  Port=23
  TMY1 : Inport  Port=24
  IPL2 : Inport  Port=25
  IPT2 : Inport  Port=26
  IPY2 : Inport  Port=27
  BFL2 : Inport  Port=28
  BFT2 : Inport  Port=29
  BFV2 : Inport  Port=30
  BFR2 : Inport  Port=31
  BFP2 : Inport  Port=32
  BFY2 : Inport  Port=33
  MNL2 : Inport  Port=34
  MNT2 : Inport  Port=35
  MNV2 : Inport  Port=36
  MNR2 : Inport  Port=37
  MNP2 : Inport  Port=38
  MNY2 : Inport  Port=39
  IML2 : Inport  Port=40
  IMT2 : Inport  Port=41
  IMV2 : Inport  Port=42
  IMR2 : Inport  Port=43
  IMP2 : Inport  Port=44
  IMY2 : Inport  Port=45
  TML2 : Inport  Port=46
  TMP2 : Inport  Port=47
  TMY2 : Inport  Port=48
  IPL3 : Inport  Port=49
  IPT3 : Inport  Port=50
  IPY3 : Inport  Port=51
  BFL3 : Inport  Port=52
  BFT3 : Inport  Port=53
  BFV3 : Inport  Port=54
  BFR3 : Inport  Port=55
  BFP3 : Inport  Port=56
  BFY3 : Inport  Port=57
  MNL3 : Inport  Port=58
  MNT3 : Inport  Port=59
  MNV3 : Inport  Port=60
  MNR3 : Inport  Port=61
  MNP3 : Inport  Port=62
  MNY3 : Inport  Port=63
  IML3 : Inport  Port=64
  IMT3 : Inport  Port=65
  IMV3 : Inport  Port=66
  IMR3 : Inport  Port=67
  IMP3 : Inport  Port=68
  IMY3 : Inport  Port=69
  TML3 : Inport  Port=70
  TMP3 : Inport  Port=71
  TMY3 : Inport  Port=72
  IPL4 : Inport  Port=73
  IPT4 : Inport  Port=74
  IPY4 : Inport  Port=75
  BFL4 : Inport  Port=76
  BFT4 : Inport  Port=77
  BFV4 : Inport  Port=78
  BFR4 : Inport  Port=79
  BFP4 : Inport  Port=80
  BFY4 : Inport  Port=81
  MNL4 : Inport  Port=82
  MNT4 : Inport  Port=83
  MNV4 : Inport  Port=84
  MNR4 : Inport  Port=85
  MNP4 : Inport  Port=86
  MNY4 : Inport  Port=87
  IML4 : Inport  Port=88
  IMT4 : Inport  Port=89
  IMV4 : Inport  Port=90
  IMR4 : Inport  Port=91
  IMP4 : Inport  Port=92
  IMY4 : Inport  Port=93
  TML4 : Inport  Port=94
  TMP4 : Inport  Port=95
  TMY4 : Inport  Port=96
  IPL5 : Inport  Port=97
  IPT5 : Inport  Port=98
  IPY5 : Inport  Port=99
  BFL5 : Inport  Port=100
  BFT5 : Inport  Port=101
  BFV5 : Inport  Port=102
  BFR5 : Inport  Port=103
  BFP5 : Inport  Port=104
  BFY5 : Inport  Port=105
  MNL5 : Inport  Port=106
  MNT5 : Inport  Port=107
  MNV5 : Inport  Port=108
  MNR5 : Inport  Port=109
  MNP5 : Inport  Port=110
  MNY5 : Inport  Port=111
  IML5 : Inport  Port=112
  IMT5 : Inport  Port=113
  IMV5 : Inport  Port=114
  IMR5 : Inport  Port=115
  IMP5 : Inport  Port=116
  IMY5 : Inport  Port=117
  TML5 : Inport  Port=118
  TMP5 : Inport  Port=119
  TMY5 : Inport  Port=120
  IPL6 : Inport  Port=121
  IPT6 : Inport  Port=122
  IPY6 : Inport  Port=123
  BFL6 : Inport  Port=124
  BFT6 : Inport  Port=125
  BFV6 : Inport  Port=126
  BFR6 : Inport  Port=127
  BFP6 : Inport  Port=128
  BFY6 : Inport  Port=129
  MNL6 : Inport  Port=130
  MNT6 : Inport  Port=131
  MNV6 : Inport  Port=132
  MNR6 : Inport  Port=133
  MNP6 : Inport  Port=134
  MNY6 : Inport  Port=135
  IML6 : Inport  Port=136
  IMT6 : Inport  Port=137
  IMV6 : Inport  Port=138
  IMR6 : Inport  Port=139
  IMP6 : Inport  Port=140
  IMY6 : Inport  Port=141
  TML6 : Inport  Port=142
  TMP6 : Inport  Port=143
  TMY6 : Inport  Port=144
  IPL7 : Inport  Port=145
  IPT7 : Inport  Port=146
  IPY7 : Inport  Port=147
  BFL7 : Inport  Port=148
  BFT7 : Inport  Port=149
  BFV7 : Inport  Port=150
  BFR7 : Inport  Port=151
  BFP7 : Inport  Port=152
  BFY7 : Inport  Port=153
  MNL7 : Inport  Port=154
  MNT7 : Inport  Port=155
  MNV7 : Inport  Port=156
  MNR7 : Inport  Port=157
  MNP7 : Inport  Port=158
  MNY7 : Inport  Port=159
  IML7 : Inport  Port=160
  IMT7 : Inport  Port=161
  IMV7 : Inport  Port=162
  IMR7 : Inport  Port=163
  IMP7 : Inport  Port=164
  IMY7 : Inport  Port=165
  TML7 : Inport  Port=166
  TMP7 : Inport  Port=167
  TMY7 : Inport  Port=168
  IPL8 : Inport  Port=169
  IPT8 : Inport  Port=170
  IPY8 : Inport  Port=171
  BFL8 : Inport  Port=172
  BFT8 : Inport  Port=173
  BFV8 : Inport  Port=174
  BFR8 : Inport  Port=175
  BFP8 : Inport  Port=176
  BFY8 : Inport  Port=177
  MNL8 : Inport  Port=178
  MNT8 : Inport  Port=179
  MNV8 : Inport  Port=180
  MNR8 : Inport  Port=181
  MNP8 : Inport  Port=182
  MNY8 : Inport  Port=183
  IML8 : Inport  Port=184
  IMT8 : Inport  Port=185
  IMV8 : Inport  Port=186
  IMR8 : Inport  Port=187
  IMP8 : Inport  Port=188
  IMY8 : Inport  Port=189
  TML8 : Inport  Port=190
  TMP8 : Inport  Port=191
  TMY8 : Inport  Port=192
  IPL9 : Inport  Port=193
  IPT9 : Inport  Port=194
  IPY9 : Inport  Port=195
  BFL9 : Inport  Port=196
  BFT9 : Inport  Port=197
  BFV9 : Inport  Port=198
  BFR9 : Inport  Port=199
  BFP9 : Inport  Port=200
  BFY9 : Inport  Port=201
  MNL9 : Inport  Port=202
  MNT9 : Inport  Port=203
  MNV9 : Inport  Port=204
  MNR9 : Inport  Port=205
  MNP9 : Inport  Port=206
  MNY9 : Inport  Port=207
  IML9 : Inport  Port=208
  IMT9 : Inport  Port=209
  IMV9 : Inport  Port=210
  IMR9 : Inport  Port=211
  IMP9 : Inport  Port=212
  IMY9 : Inport  Port=213
  TML9 : Inport  Port=214
  TMP9 : Inport  Port=215
  TMY9 : Inport  Port=216
  IPL10 : Inport  Port=217
  IPT10 : Inport  Port=218
  IPY10 : Inport  Port=219
  BFL10 : Inport  Port=220
  BFT10 : Inport  Port=221
  BFV10 : Inport  Port=222
  BFR10 : Inport  Port=223
  BFP10 : Inport  Port=224
  BFY10 : Inport  Port=225
  MNL10 : Inport  Port=226
  MNT10 : Inport  Port=227
  MNV10 : Inport  Port=228
  MNR10 : Inport  Port=229
  MNP10 : Inport  Port=230
  MNY10 : Inport  Port=231
  IML10 : Inport  Port=232
  IMT10 : Inport  Port=233
  IMV10 : Inport  Port=234
  IMR10 : Inport  Port=235
  IMP10 : Inport  Port=236
  IMY10 : Inport  Port=237
  TML10 : Inport  Port=238
  TMP10 : Inport  Port=239
  TMY10 : Inport  Port=240
  IPL11 : Inport  Port=241
  IPT11 : Inport  Port=242
  IPY11 : Inport  Port=243
  BFL11 : Inport  Port=244
  BFT11 : Inport  Port=245
  BFV11 : Inport  Port=246
  BFR11 : Inport  Port=247
  BFP11 : Inport  Port=248
  BFY11 : Inport  Port=249
  MNL11 : Inport  Port=250
  MNT11 : Inport  Port=251
  MNV11 : Inport  Port=252
  MNR11 : Inport  Port=253
  MNP11 : Inport  Port=254
  MNY11 : Inport  Port=255
  IML11 : Inport  Port=256
  IMT11 : Inport  Port=257
  IMV11 : Inport  Port=258
  IMR11 : Inport  Port=259
  IMP11 : Inport  Port=260
  IMY11 : Inport  Port=261
  TML11 : Inport  Port=262
  TMP11 : Inport  Port=263
  TMY11 : Inport  Port=264
  IPL12 : Inport  Port=265
  IPT12 : Inport  Port=266
  IPY12 : Inport  Port=267
  BFL12 : Inport  Port=268
  BFT12 : Inport  Port=269
  BFV12 : Inport  Port=270
  BFR12 : Inport  Port=271
  BFP12 : Inport  Port=272
  BFY12 : Inport  Port=273
  MNL12 : Inport  Port=274
  MNT12 : Inport  Port=275
  MNV12 : Inport  Port=276
  MNR12 : Inport  Port=277
  MNP12 : Inport  Port=278
  MNY12 : Inport  Port=279
  IML12 : Inport  Port=280
  IMT12 : Inport  Port=281
  IMV12 : Inport  Port=282
  IMR12 : Inport  Port=283
  IMP12 : Inport  Port=284
  IMY12 : Inport  Port=285
  TML12 : Inport  Port=286
  TMP12 : Inport  Port=287
  TMY12 : Inport  Port=288
  sum{1..24} (24 alike) : VIS_LIB/MODAL/sum
  IPL : Outport
  IPT : Outport  Port=2
  IPY : Outport  Port=3
  BFL : Outport  Port=4
  BFT : Outport  Port=5
  BFV : Outport  Port=6
  BFR : Outport  Port=7
  BFP : Outport  Port=8
  BFY : Outport  Port=9
  MNL : Outport  Port=10
  MNT : Outport  Port=11
  MNV : Outport  Port=12
  MNR : Outport  Port=13
  MNP : Outport  Port=14
  MNY : Outport  Port=15
  IML : Outport  Port=16
  IMT : Outport  Port=17
  IMV : Outport  Port=18
  IMR : Outport  Port=19
  IMP : Outport  Port=20
  IMY : Outport  Port=21
  TML : Outport  Port=22
  TMP : Outport  Port=23
  TMY : Outport  Port=24
  wires:
  IPT2/1 -> sum1/2
  IPT1/1 -> sum1/1
  IPL1/1 -> sum2/1
  IPL2/1 -> sum2/2
  IPY1/1 -> sum3/1
  IPY2/1 -> sum3/2
  BFT1/1 -> sum4/1
  BFT2/1 -> sum4/2
  BFL1/1 -> sum5/1
  BFL2/1 -> sum5/2
  BFV1/1 -> sum6/1
  BFV2/1 -> sum6/2
  BFR1/1 -> sum8/1
  BFR2/1 -> sum8/2
  BFP1/1 -> sum7/1
  BFP2/1 -> sum7/2
  BFY1/1 -> sum9/1
  BFY2/1 -> sum9/2
  MNT1/1 -> sum10/1
  MNT2/1 -> sum10/2
  MNL1/1 -> sum11/1
  MNL2/1 -> sum11/2
  MNV1/1 -> sum12/1
  MNV2/1 -> sum12/2
  MNR1/1 -> sum14/1
  MNR2/1 -> sum14/2
  MNP1/1 -> sum13/1
  MNP2/1 -> sum13/2
  MNY1/1 -> sum15/1
  MNY2/1 -> sum15/2
  IMT1/1 -> sum16/1
  IMT2/1 -> sum16/2
  IML1/1 -> sum17/1
  IML2/1 -> sum17/2
  IMV1/1 -> sum18/1
  IMV2/1 -> sum18/2
  IMP1/1 -> sum19/1
  IMP2/1 -> sum19/2
  IMY1/1 -> sum21/1
  IMY2/1 -> sum21/2
  TML2/1 -> sum23/2
  TML1/1 -> sum23/1
  TMP1/1 -> sum22/1
  TMP2/1 -> sum22/2
  TMY1/1 -> sum24/1
  TMY2/1 -> sum24/2
  sum24/1 -> TMY/1
  sum22/1 -> TMP/1
  sum23/1 -> TML/1
  sum17/1 -> IML/1
  sum16/1 -> IMT/1
  sum18/1 -> IMV/1
  sum20/1 -> IMR/1
  sum19/1 -> IMP/1
  sum21/1 -> IMY/1
  sum3/1 -> IPY/1
  sum1/1 -> IPT/1
  sum4/1 -> BFT/1
  sum6/1 -> BFV/1
  sum12/1 -> MNV/1
  sum14/1 -> MNR/1
  sum8/1 -> BFR/1
  sum7/1 -> BFP/1
  sum9/1 -> BFY/1
  sum15/1 -> MNY/1
  sum13/1 -> MNP/1
  sum10/1 -> MNT/1
  sum11/1 -> MNL/1
  sum5/1 -> BFL/1
  sum2/1 -> IPL/1
  IPT3/1 -> sum1/3
  IPL3/1 -> sum2/3
  IPY3/1 -> sum3/3
  BFT3/1 -> sum4/3
  BFL3/1 -> sum5/3
  BFV3/1 -> sum6/3
  BFR3/1 -> sum8/3
  BFP3/1 -> sum7/3
  BFY3/1 -> sum9/3
  MNT3/1 -> sum10/3
  MNL3/1 -> sum11/3
  MNV3/1 -> sum12/3
  MNR3/1 -> sum14/3
  MNP3/1 -> sum13/3
  MNY3/1 -> sum15/3
  IMT3/1 -> sum16/3
  IML3/1 -> sum17/3
  IMV3/1 -> sum18/3
  IMP3/1 -> sum19/3
  IMY3/1 -> sum21/3
  TML3/1 -> sum23/3
  TMP3/1 -> sum22/3
  TMY3/1 -> sum24/3
  IPT4/1 -> sum1/4
  IPL4/1 -> sum2/4
  IPY4/1 -> sum3/4
  BFT4/1 -> sum4/4
  BFL4/1 -> sum5/4
  BFV4/1 -> sum6/4
  BFR4/1 -> sum8/4
  BFP4/1 -> sum7/4
  BFY4/1 -> sum9/4
  MNT4/1 -> sum10/4
  MNL4/1 -> sum11/4
  MNV4/1 -> sum12/4
  MNR4/1 -> sum14/4
  MNP4/1 -> sum13/4
  MNY4/1 -> sum15/4
  IMT4/1 -> sum16/4
  IML4/1 -> sum17/4
  IMV4/1 -> sum18/4
  IMP4/1 -> sum19/4
  IMY4/1 -> sum21/4
  TML4/1 -> sum23/4
  TMP4/1 -> sum22/4
  TMY4/1 -> sum24/4
  IPT5/1 -> sum1/5
  IPL5/1 -> sum2/5
  IPY5/1 -> sum3/5
  BFT5/1 -> sum4/5
  BFL5/1 -> sum5/5
  BFV5/1 -> sum6/5
  BFR5/1 -> sum8/5
  BFP5/1 -> sum7/5
  BFY5/1 -> sum9/5
  MNT5/1 -> sum10/5
  MNL5/1 -> sum11/5
  MNV5/1 -> sum12/5
  MNR5/1 -> sum14/5
  MNP5/1 -> sum13/5
  MNY5/1 -> sum15/5
  IMT5/1 -> sum16/5
  IML5/1 -> sum17/5
  IMV5/1 -> sum18/5
  IMP5/1 -> sum19/5
  IMY5/1 -> sum21/5
  TML5/1 -> sum23/5
  TMP5/1 -> sum22/5
  TMY5/1 -> sum24/5
  IPT6/1 -> sum1/6
  IPL6/1 -> sum2/6
  IPY6/1 -> sum3/6
  BFT6/1 -> sum4/6
  BFL6/1 -> sum5/6
  BFV6/1 -> sum6/6
  BFR6/1 -> sum8/6
  BFP6/1 -> sum7/6
  BFY6/1 -> sum9/6
  MNT6/1 -> sum10/6
  MNL6/1 -> sum11/6
  MNV6/1 -> sum12/6
  MNR6/1 -> sum14/6
  MNP6/1 -> sum13/6
  MNY6/1 -> sum15/6
  IMT6/1 -> sum16/6
  IML6/1 -> sum17/6
  IMV6/1 -> sum18/6
  IMP6/1 -> sum19/6
  IMY6/1 -> sum21/6
  TML6/1 -> sum23/6
  TMP6/1 -> sum22/6
  TMY6/1 -> sum24/6
  IPT7/1 -> sum1/7
  IPL7/1 -> sum2/7
  IPY7/1 -> sum3/7
  BFT7/1 -> sum4/7
  BFL7/1 -> sum5/7
  BFV7/1 -> sum6/7
  BFR7/1 -> sum8/7
  BFP7/1 -> sum7/7
  BFY7/1 -> sum9/7
  MNT7/1 -> sum10/7
  MNL7/1 -> sum11/7
  MNV7/1 -> sum12/7
  MNR7/1 -> sum14/7
  MNP7/1 -> sum13/7
  MNY7/1 -> sum15/7
  IMT7/1 -> sum16/7
  IML7/1 -> sum17/7
  IMV7/1 -> sum18/7
  IMP7/1 -> sum19/7
  IMY7/1 -> sum21/7
  TML7/1 -> sum23/7
  TMP7/1 -> sum22/7
  TMY7/1 -> sum24/7
  IPT8/1 -> sum1/8
  IPL8/1 -> sum2/8
  IPY8/1 -> sum3/8
  BFT8/1 -> sum4/8
  BFL8/1 -> sum5/8
  BFV8/1 -> sum6/8
  BFR8/1 -> sum8/8
  BFP8/1 -> sum7/8
  BFY8/1 -> sum9/8
  MNT8/1 -> sum10/8
  MNL8/1 -> sum11/8
  MNV8/1 -> sum12/8
  MNR8/1 -> sum14/8
  MNP8/1 -> sum13/8
  MNY8/1 -> sum15/8
  IMT8/1 -> sum16/8
  IML8/1 -> sum17/8
  IMV8/1 -> sum18/8
  IMP8/1 -> sum19/8
  IMY8/1 -> sum21/8
  TML8/1 -> sum23/8
  TMP8/1 -> sum22/8
  TMY8/1 -> sum24/8
  IPT9/1 -> sum1/9
  IPL9/1 -> sum2/9
  IPY9/1 -> sum3/9
  BFT9/1 -> sum4/9
  BFL9/1 -> sum5/9
  BFV9/1 -> sum6/9
  BFR9/1 -> sum8/9
  BFP9/1 -> sum7/9
  BFY9/1 -> sum9/9
  MNT9/1 -> sum10/9
  MNL9/1 -> sum11/9
  MNV9/1 -> sum12/9
  MNR9/1 -> sum14/9
  MNP9/1 -> sum13/9
  MNY9/1 -> sum15/9
  IMT9/1 -> sum16/9
  IML9/1 -> sum17/9
  IMV9/1 -> sum18/9
  IMP9/1 -> sum19/9
  IMY9/1 -> sum21/9
  TML9/1 -> sum23/9
  TMP9/1 -> sum22/9
  TMY9/1 -> sum24/9
  IPT10/1 -> sum1/10
  IPL10/1 -> sum2/10
  IPY10/1 -> sum3/10
  BFT10/1 -> sum4/10
  BFL10/1 -> sum5/10
  BFV10/1 -> sum6/10
  BFR10/1 -> sum8/10
  BFP10/1 -> sum7/10
  BFY10/1 -> sum9/10
  MNT10/1 -> sum10/10
  MNL10/1 -> sum11/10
  MNV10/1 -> sum12/10
  MNR10/1 -> sum14/10
  MNP10/1 -> sum13/10
  MNY10/1 -> sum15/10
  IMT10/1 -> sum16/10
  IML10/1 -> sum17/10
  IMV10/1 -> sum18/10
  IMP10/1 -> sum19/10
  IMY10/1 -> sum21/10
  TML10/1 -> sum23/10
  TMP10/1 -> sum22/10
  TMY10/1 -> sum24/10
  IPT11/1 -> sum1/11
  IPL11/1 -> sum2/11
  IPY11/1 -> sum3/11
  BFT11/1 -> sum4/11
  BFL11/1 -> sum5/11
  BFV11/1 -> sum6/11
  BFR11/1 -> sum8/11
  BFP11/1 -> sum7/11
  BFY11/1 -> sum9/11
  MNT11/1 -> sum10/11
  MNL11/1 -> sum11/11
  MNV11/1 -> sum12/11
  MNR11/1 -> sum14/11
  MNP11/1 -> sum13/11
  MNY11/1 -> sum15/11
  IMT11/1 -> sum16/11
  IML11/1 -> sum17/11
  IMV11/1 -> sum18/11
  IMP11/1 -> sum19/11
  IMY11/1 -> sum21/11
  TML11/1 -> sum23/11
  TMP11/1 -> sum22/11
  TMY11/1 -> sum24/11
  IPT12/1 -> sum1/12
  IPL12/1 -> sum2/12
  IPY12/1 -> sum3/12
  BFT12/1 -> sum4/12
  BFL12/1 -> sum5/12
  BFV12/1 -> sum6/12
  BFR12/1 -> sum8/12
  BFP12/1 -> sum7/12
  BFY12/1 -> sum9/12
  MNT12/1 -> sum10/12
  MNL12/1 -> sum11/12
  MNV12/1 -> sum12/12
  MNR12/1 -> sum14/12
  MNP12/1 -> sum13/12
  MNY12/1 -> sum15/12
  IMT12/1 -> sum16/12
  IML12/1 -> sum17/12
  IMV12/1 -> sum18/12
  IMP12/1 -> sum19/12
  IMY12/1 -> sum21/12
  TML12/1 -> sum23/12
  TMP12/1 -> sum22/12
  TMY12/1 -> sum24/12
  IMR12/1 -> sum20/12
  IMR11/1 -> sum20/11
  IMR10/1 -> sum20/10
  IMR9/1 -> sum20/9
  IMR8/1 -> sum20/8
  IMR7/1 -> sum20/7
  IMR6/1 -> sum20/6
  IMR5/1 -> sum20/5
  IMR4/1 -> sum20/4
  IMR3/1 -> sum20/3
  IMR2/1 -> sum20/2
  IMR1/1 -> sum20/1

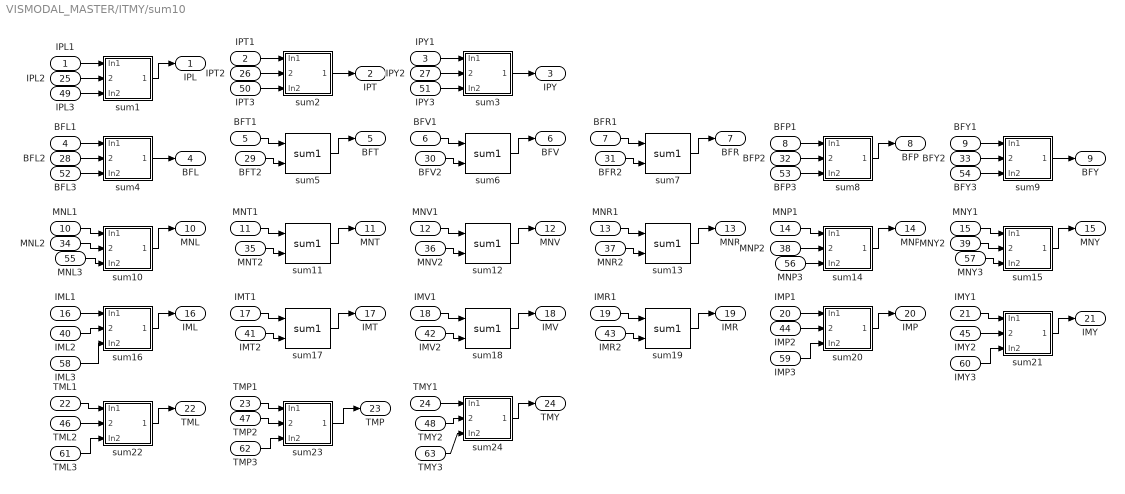
== system VISMODAL_MASTER/ITMY/sum10 ==
  IPL1 : Inport
  IPT1 : Inport  Port=2
  IPY1 : Inport  Port=3
  BFL1 : Inport  Port=4
  BFT1 : Inport  Port=5
  BFV1 : Inport  Port=6
  BFR1 : Inport  Port=7
  BFP1 : Inport  Port=8
  BFY1 : Inport  Port=9
  MNL1 : Inport  Port=10
  MNT1 : Inport  Port=11
  MNV1 : Inport  Port=12
  MNR1 : Inport  Port=13
  MNP1 : Inport  Port=14
  MNY1 : Inport  Port=15
  IML1 : Inport  Port=16
  IMT1 : Inport  Port=17
  IMV1 : Inport  Port=18
  IMR1 : Inport  Port=19
  IMP1 : Inport  Port=20
  IMY1 : Inport  Port=21
  TML1 : Inport  Port=22
  TMP1 : Inport  Port=23
  TMY1 : Inport  Port=24
  IPL2 : Inport  Port=25
  IPT2 : Inport  Port=26
  IPY2 : Inport  Port=27
  BFL2 : Inport  Port=28
  BFT2 : Inport  Port=29
  BFV2 : Inport  Port=30
  BFR2 : Inport  Port=31
  BFP2 : Inport  Port=32
  BFY2 : Inport  Port=33
  MNL2 : Inport  Port=34
  MNT2 : Inport  Port=35
  MNV2 : Inport  Port=36
  MNR2 : Inport  Port=37
  MNP2 : Inport  Port=38
  MNY2 : Inport  Port=39
  IML2 : Inport  Port=40
  IMT2 : Inport  Port=41
  IMV2 : Inport  Port=42
  IMR2 : Inport  Port=43
  IMP2 : Inport  Port=44
  IMY2 : Inport  Port=45
  TML2 : Inport  Port=46
  TMP2 : Inport  Port=47
  TMY2 : Inport  Port=48
  IPL3 : Inport  Port=49
  IPT3 : Inport  Port=50
  IPY3 : Inport  Port=51
  BFL3 : Inport  Port=52
  BFP3 : Inport  Port=53
  BFY3 : Inport  Port=54
  MNL3 : Inport  Port=55
  MNP3 : Inport  Port=56
  MNY3 : Inport  Port=57
  IML3 : Inport  Port=58
  IMP3 : Inport  Port=59
  IMY3 : Inport  Port=60
  TML3 : Inport  Port=61
  TMP3 : Inport  Port=62
  TMY3 : Inport  Port=63
  sum1 : Subsystem
  sum10 : Subsystem
  sum{5..7,11..13,17..19} (9 alike) : VIS_LIB/MODAL/sum1
  sum14 : Subsystem
  sum15 : Subsystem
  sum16 : Subsystem
  sum2 : Subsystem
  sum20 : Subsystem
  sum21 : Subsystem
  sum22 : Subsystem
  sum23 : Subsystem
  sum24 : Subsystem
  sum3 : Subsystem
  sum4 : Subsystem
  sum8 : Subsystem
  sum9 : Subsystem
  IPL : Outport
  IPT : Outport  Port=2
  IPY : Outport  Port=3
  BFL : Outport  Port=4
  BFT : Outport  Port=5
  BFV : Outport  Port=6
  BFR : Outport  Port=7
  BFP : Outport  Port=8
  BFY : Outport  Port=9
  MNL : Outport  Port=10
  MNT : Outport  Port=11
  MNV : Outport  Port=12
  MNR : Outport  Port=13
  MNP : Outport  Port=14
  MNY : Outport  Port=15
  IML : Outport  Port=16
  IMT : Outport  Port=17
  IMV : Outport  Port=18
  IMR : Outport  Port=19
  IMP : Outport  Port=20
  IMY : Outport  Port=21
  TML : Outport  Port=22
  TMP : Outport  Port=23
  TMY : Outport  Port=24
  wires:
  sum1/1(Out1) -> IPL/1
  IPL1/1 -> sum1/1(In1)
  sum2/1(Out1) -> IPT/1
  IPT1/1 -> sum2/1(In1)
  BFL1/1 -> sum4/1(In1)
  sum5/1 -> BFT/1
  BFT1/1 -> sum5/1
  sum6/1 -> BFV/1
  BFV1/1 -> sum6/1
  sum7/1 -> BFR/1
  BFR1/1 -> sum7/1
  sum8/1(Out1) -> BFP/1
  BFP1/1 -> sum8/1(In1)
  sum9/1(Out1) -> BFY/1
  BFY1/1 -> sum9/1(In1)
  sum10/1(Out1) -> MNL/1
  MNL1/1 -> sum10/1(In1)
  sum11/1 -> MNT/1
  MNT1/1 -> sum11/1
  sum12/1 -> MNV/1
  MNV1/1 -> sum12/1
  sum13/1 -> MNR/1
  MNR1/1 -> sum13/1
  sum14/1(Out1) -> MNP/1
  MNP1/1 -> sum14/1(In1)
  sum15/1(Out1) -> MNY/1
  MNY1/1 -> sum15/1(In1)
  sum16/1(Out1) -> IML/1
  IML1/1 -> sum16/1(In1)
  sum17/1 -> IMT/1
  IMT1/1 -> sum17/1
  sum18/1 -> IMV/1
  IMV1/1 -> sum18/1
  sum19/1 -> IMR/1
  IMR1/1 -> sum19/1
  sum20/1(Out1) -> IMP/1
  IMP1/1 -> sum20/1(In1)
  sum21/1(Out1) -> IMY/1
  IMY1/1 -> sum21/1(In1)
  sum22/1(Out1) -> TML/1
  TML1/1 -> sum22/1(In1)
  sum23/1(Out1) -> TMP/1
  TMP1/1 -> sum23/1(In1)
  sum24/1(Out1) -> TMY/1
  TMY1/1 -> sum24/1(In1)
  IPL2/1 -> sum1/2(In12)
  IPT2/1 -> sum2/2(In12)
  BFT2/1 -> sum5/2
  BFV2/1 -> sum6/2
  BFR2/1 -> sum7/2
  BFY2/1 -> sum9/2(In12)
  MNL2/1 -> sum10/2(In12)
  MNT2/1 -> sum11/2
  MNV2/1 -> sum12/2
  MNR2/1 -> sum13/2
  MNY2/1 -> sum15/2(In12)
  IML2/1 -> sum16/2(In12)
  IMT2/1 -> sum17/2
  IMV2/1 -> sum18/2
  IMR2/1 -> sum19/2
  IMP2/1 -> sum20/2(In12)
  TMP2/1 -> sum23/2(In12)
  TMY2/1 -> sum24/2(In12)
  sum4/1(Out1) -> BFL/1
  BFL2/1 -> sum4/2(In12)
  BFP2/1 -> sum8/2(In12)
  MNP2/1 -> sum14/2(In12)
  BFY3/1 -> sum9/3(In2)
  BFL3/1 -> sum4/3(In2)
  BFP3/1 -> sum8/3(In2)
  MNL3/1 -> sum10/3(In2)
  MNY3/1 -> sum15/3(In2)
  MNP3/1 -> sum14/3(In2)
  IPY1/1 -> sum3/1(In1)
  IPY2/1 -> sum3/2(In12)
  sum3/1(Out1) -> IPY/1
  IPL3/1 -> sum1/3(In2)
  IPT3/1 -> sum2/3(In2)
  IPY3/1 -> sum3/3(In2)
  TML2/1 -> sum22/2(In12)
  IMY2/1 -> sum21/2(In12)
  IML3/1 -> sum16/3(In2)
  TML3/1 -> sum22/3(In2)
  TMP3/1 -> sum23/3(In2)
  TMY3/1 -> sum24/3(In2)
  IMP3/1 -> sum20/3(In2)
  IMY3/1 -> sum21/3(In2)
